simulink library "carnotUIBK_bus"  (R2023b)
settings: Solver=VariableStepAuto  StartTime=0.0  StopTime=10.0  RelTol=1e-3  EnableMultiTasking=on
values from neighbouring files (symbols this model uses):
  A = 7*10*2    (= 140)    [theta_ground_v1.m]    (also in xlswrite1.m = num2cell(data))
  amb_factor = 1    [DOOR.m]    (also in WALL.m; WINDOW.m = 0)
  area = obj.width * obj.height    [DOOR.m]    (also in RES.m = []; ROOM.m = 0; THERMALZONE.m = area + room(kk).area; WALL.m = area - obj.doors(jj).calc_area())
  B = A/(0.5 * P)    (= 8.23529411765)    [theta_ground_v1.m]
  boundary = BOUNDARY()    [BUILDING.m]    (also in WALL.m = '')
  building = obj    [BUILDING.m]    (also in create_building_automatic.m = building.save(); ini_building_automatic.m = building.add_variant_hvac(building.variant_hvac, hvac); load_building_automatic.m = building.save())
  C = zeros(1,length(d)+1)    [CONSTRUCTION.m]    (also in DOOR.m = [0 0 0]; WALL.m = [0 0 0]; WINDOW.m = [0 0 0])
  control = 2    [GAIN.m]    (also in GAINS.m)
  cp = str2num(value)    [CONSTRUCTION.m]
  height = 0    [DOOR.m]    (also in ROOM.m; THERMALZONE.m; WALL.m; WINDOW.m)
  p = [timevec_weather weather(:,12)]    [BOUNDARY.m]    (also in WEATHER.m = 0; init_carnotUIBK.m = cell2mat(carnotUIBKpaths(i,2)))
  rho = str2num(value)    [CONSTRUCTION.m]    (also in theta_ground_v1.m = 2000)
  type = 1    [CONSTRUCTION.m]    (also in GAINS.m = raw_moisture{ii,3}; STRUCTURE.m = 0)
  view_factor = 1    [DOOR.m]    (also in WINDOW.m = 0)
  wall = []    [ROOM.m]
  z = obj.Z    [WALL.m]    (also in theta_ground_v1.m = 0)
  zone = obj.zone(ind)    [THERMALZONE.m]
undefined symbols (not defined in the file or in its folder): const, Dd, get_building, mdot_air, mdot_CO2, mdot_H2O, mdot_VOC, pos, Qdot_C, Qdot_H, Qdot_I_electricity, Qdot_I_light, Qdot_I_person, Qdot_S, Qdot_T_ground, Qdot_T_internal, Qdot_T_neighbour, Qdot_T_opaque, Qdot_T_window, Qdot_V_infiltration, Qdot_V_mech, Qdot_V_window, Qdotc, Qdotr, r_frame, solar_ratio, solar_ratio1, solar_ratio2, Tc, Tr, Ts, Uvalue, wallsurface, window, window_height, window_heigth, window_width, windowsurface, x_CO2, x_H2O, x_VOC
libraries: $bdroot x134, carnot x87, simulink_extras x14, slpidlib x4, simulink x3
(part 5 of 12)

== system carnotUIBK_bus/HVAC/HVAC_9002_window opening/window opening 2 ==
  setpoint : Inport
  AIB : Inport  Port=2
  WDB : Inport  Port=3
  Enable : EnablePort
  Add : Sum
  Bus Selector1 : BusSelector  OutputSignals=Temperature_Ambient
  Bus Selector5 : BusSelector  OutputSignals=Ts,Tc,p,x_H2O
  Product : Product
  Saturation : Saturate  UpperLimit=1  LowerLimit=0
  Sum : Sum  Inputs=|-+
  Sum1 : Sum  Inputs=|+-
  Sum2 : Sum  Inputs=|-+
  Transfer Fcn (with initial states)1 : Subsystem  mask(Transfer Function with Initial States){N=[1], D=[600 1], X0=0}
      mask prompts: N "Numerator:"; D "Denominator:"; X0 "Initial conditions:"
      mask help: Vector expressions for numerator, and denominator. Coefficients are in descending powers of s.
      mask init:
      | [A,B,C,Dd]=tf2ss(N,D);if (isempty(X0));[m,n]=size(A);X0=zeros(1,m); end;
      mask Help: Specify the initial states for the transfer function.  The state ordering is determined by the m-file tf2ss.  There is no unique mapping of the states in a transfer function to states in a state-space representation.  However, tf2ss will consistently use the same mapping for a given transfer function.
      mask Display: dpoly(N,D,'s')
  Transfer Fcn (with initial states)2 : Subsystem  mask(Transfer Function with Initial States){N=[1], D=[600 1], X0=0}
      mask prompts: N "Numerator:"; D "Denominator:"; X0 "Initial conditions:"
      mask help: Vector expressions for numerator, and denominator. Coefficients are in descending powers of s.
      mask init:
      | [A,B,C,Dd]=tf2ss(N,D);if (isempty(X0));[m,n]=size(A);X0=zeros(1,m); end;
      mask Help: Specify the initial states for the transfer function.  The state ordering is determined by the m-file tf2ss.  There is no unique mapping of the states in a transfer function to states in a state-space representation.  However, tf2ss will consistently use the same mapping for a given transfer function.
      mask Display: dpoly(N,D,'s')
  Transfer Fcn (with initial states)3 : Subsystem  mask(Transfer Function with Initial States){N=[1], D=[600 1], X0=0}
      mask prompts: N "Numerator:"; D "Denominator:"; X0 "Initial conditions:"
      mask help: Vector expressions for numerator, and denominator. Coefficients are in descending powers of s.
      mask init:
      | [A,B,C,Dd]=tf2ss(N,D);if (isempty(X0));[m,n]=size(A);X0=zeros(1,m); end;
      mask Help: Specify the initial states for the transfer function.  The state ordering is determined by the m-file tf2ss.  There is no unique mapping of the states in a transfer function to states in a state-space representation.  However, tf2ss will consistently use the same mapping for a given transfer function.
      mask Display: dpoly(N,D,'s')
  on/off ambient : Relay  OnSwitchValue=0.5  OffSwitchValue=-0.5
  on/off hum : Relay  OnSwitchValue=0.5  OffSwitchValue=-0.5
  on/off roomtemp : Relay  OnSwitchValue=0.5  OffSwitchValue=-0.5
  setpoint humidity : Constant  Value=85
  x2RelHum_UIBK : carnot/Basic/Material_Properties/x2RelHum
      settings: SourceProductName=Carnot
  state : Outport  VectorParamsAs1DForOutWhenUnconnected=off
  wires:
  Transfer Fcn (with initial states)1/1(Out1) -> Sum2/2
  Transfer Fcn (with initial states)3/1(Out1) -> Sum1/2
  Transfer Fcn (with initial states)2/1(Out1) -> Sum/2, Sum1/1
  Saturation/1 -> state/1
  on/off hum/1 -> Add/1
  Product/1 -> Add/2
  Add/1 -> Saturation/1
  setpoint humidity/1 -> Sum2/1
  x2RelHum_UIBK/1 -> Transfer Fcn (with initial states)1/1(In1)
  Sum2/1 -> on/off hum/1
  Bus Selector5/4 -> x2RelHum_UIBK/3  "<x_H2O>"
  Bus Selector5/3 -> x2RelHum_UIBK/2  "<p>"
  Bus Selector5/2 -> x2RelHum_UIBK/1  "<Tc>"
  on/off ambient/1 -> Product/2
  Sum1/1 -> on/off ambient/1
  Bus Selector1/1 -> Transfer Fcn (with initial states)3/1(In1)  "<Temperature_Ambient>"
  WDB/1 -> Bus Selector1/1
  on/off roomtemp/1 -> Product/1
  Sum/1 -> on/off roomtemp/1
  Bus Selector5/1 -> Transfer Fcn (with initial states)2/1(In1)  "<Ts>"
  setpoint/1 -> Sum/1
  AIB/1 -> Bus Selector5/1

== system carnotUIBK_bus/HVAC/HVAC_9002_window opening/window opening 3 ==
  setpoint : Inport
  AIB : Inport  Port=2
  WDB : Inport  Port=3
  Enable : EnablePort
  Add : Sum
  Bus Selector1 : BusSelector  OutputSignals=Temperature_Ambient
  Bus Selector5 : BusSelector  OutputSignals=Ts,Tc,p,x_H2O
  Product : Product
  Saturation : Saturate  UpperLimit=1  LowerLimit=0
  Sum : Sum  Inputs=|-+
  Sum1 : Sum  Inputs=|+-
  Sum2 : Sum  Inputs=|-+
  Transfer Fcn (with initial states)1 : Subsystem  mask(Transfer Function with Initial States){N=[1], D=[600 1], X0=0}
      mask prompts: N "Numerator:"; D "Denominator:"; X0 "Initial conditions:"
      mask help: Vector expressions for numerator, and denominator. Coefficients are in descending powers of s.
      mask init:
      | [A,B,C,Dd]=tf2ss(N,D);if (isempty(X0));[m,n]=size(A);X0=zeros(1,m); end;
      mask Help: Specify the initial states for the transfer function.  The state ordering is determined by the m-file tf2ss.  There is no unique mapping of the states in a transfer function to states in a state-space representation.  However, tf2ss will consistently use the same mapping for a given transfer function.
      mask Display: dpoly(N,D,'s')
  Transfer Fcn (with initial states)2 : Subsystem  mask(Transfer Function with Initial States){N=[1], D=[600 1], X0=0}
      mask prompts: N "Numerator:"; D "Denominator:"; X0 "Initial conditions:"
      mask help: Vector expressions for numerator, and denominator. Coefficients are in descending powers of s.
      mask init:
      | [A,B,C,Dd]=tf2ss(N,D);if (isempty(X0));[m,n]=size(A);X0=zeros(1,m); end;
      mask Help: Specify the initial states for the transfer function.  The state ordering is determined by the m-file tf2ss.  There is no unique mapping of the states in a transfer function to states in a state-space representation.  However, tf2ss will consistently use the same mapping for a given transfer function.
      mask Display: dpoly(N,D,'s')
  Transfer Fcn (with initial states)3 : Subsystem  mask(Transfer Function with Initial States){N=[1], D=[600 1], X0=0}
      mask prompts: N "Numerator:"; D "Denominator:"; X0 "Initial conditions:"
      mask help: Vector expressions for numerator, and denominator. Coefficients are in descending powers of s.
      mask init:
      | [A,B,C,Dd]=tf2ss(N,D);if (isempty(X0));[m,n]=size(A);X0=zeros(1,m); end;
      mask Help: Specify the initial states for the transfer function.  The state ordering is determined by the m-file tf2ss.  There is no unique mapping of the states in a transfer function to states in a state-space representation.  However, tf2ss will consistently use the same mapping for a given transfer function.
      mask Display: dpoly(N,D,'s')
  on/off ambient : Relay  OnSwitchValue=0.5  OffSwitchValue=-0.5
  on/off hum : Relay  OnSwitchValue=0.5  OffSwitchValue=-0.5
  on/off roomtemp : Relay  OnSwitchValue=0.5  OffSwitchValue=-0.5
  setpoint humidity : Constant  Value=85
  x2RelHum_UIBK : carnot/Basic/Material_Properties/x2RelHum
      settings: SourceProductName=Carnot
  state : Outport  VectorParamsAs1DForOutWhenUnconnected=off
  wires:
  AIB/1 -> Bus Selector5/1
  setpoint/1 -> Sum/1
  Bus Selector5/1 -> Transfer Fcn (with initial states)3/1(In1)  "<Ts>"
  Sum/1 -> on/off roomtemp/1
  on/off roomtemp/1 -> Product/1
  WDB/1 -> Bus Selector1/1
  Bus Selector1/1 -> Transfer Fcn (with initial states)2/1(In1)  "<Temperature_Ambient>"
  Sum1/1 -> on/off ambient/1
  on/off ambient/1 -> Product/2
  Bus Selector5/2 -> x2RelHum_UIBK/1  "<Tc>"
  Bus Selector5/3 -> x2RelHum_UIBK/2  "<p>"
  Bus Selector5/4 -> x2RelHum_UIBK/3  "<x_H2O>"
  Sum2/1 -> on/off hum/1
  x2RelHum_UIBK/1 -> Transfer Fcn (with initial states)1/1(In1)
  setpoint humidity/1 -> Sum2/1
  Add/1 -> Saturation/1
  Product/1 -> Add/2
  on/off hum/1 -> Add/1
  Saturation/1 -> state/1
  Transfer Fcn (with initial states)3/1(Out1) -> Sum1/1, Sum/2
  Transfer Fcn (with initial states)2/1(Out1) -> Sum1/2
  Transfer Fcn (with initial states)1/1(Out1) -> Sum2/2

== system carnotUIBK_bus/HVAC/HVAC_9002_window opening/window opening 4 ==
  setpoint : Inport
  AIB : Inport  Port=2
  WDB : Inport  Port=3
  Enable : EnablePort
  Add : Sum
  Bus Selector1 : BusSelector  OutputSignals=Temperature_Ambient
  Bus Selector5 : BusSelector  OutputSignals=Ts,Tc,p,x_H2O
  Product : Product
  Saturation : Saturate  UpperLimit=1  LowerLimit=0
  Sum : Sum  Inputs=|-+
  Sum1 : Sum  Inputs=|+-
  Sum2 : Sum  Inputs=|-+
  Transfer Fcn (with initial states)1 : Subsystem  mask(Transfer Function with Initial States){N=[1], D=[600 1], X0=0}
      mask prompts: N "Numerator:"; D "Denominator:"; X0 "Initial conditions:"
      mask help: Vector expressions for numerator, and denominator. Coefficients are in descending powers of s.
      mask init:
      | [A,B,C,Dd]=tf2ss(N,D);if (isempty(X0));[m,n]=size(A);X0=zeros(1,m); end;
      mask Help: Specify the initial states for the transfer function.  The state ordering is determined by the m-file tf2ss.  There is no unique mapping of the states in a transfer function to states in a state-space representation.  However, tf2ss will consistently use the same mapping for a given transfer function.
      mask Display: dpoly(N,D,'s')
  Transfer Fcn (with initial states)2 : Subsystem  mask(Transfer Function with Initial States){N=[1], D=[600 1], X0=0}
      mask prompts: N "Numerator:"; D "Denominator:"; X0 "Initial conditions:"
      mask help: Vector expressions for numerator, and denominator. Coefficients are in descending powers of s.
      mask init:
      | [A,B,C,Dd]=tf2ss(N,D);if (isempty(X0));[m,n]=size(A);X0=zeros(1,m); end;
      mask Help: Specify the initial states for the transfer function.  The state ordering is determined by the m-file tf2ss.  There is no unique mapping of the states in a transfer function to states in a state-space representation.  However, tf2ss will consistently use the same mapping for a given transfer function.
      mask Display: dpoly(N,D,'s')
  Transfer Fcn (with initial states)3 : Subsystem  mask(Transfer Function with Initial States){N=[1], D=[600 1], X0=0}
      mask prompts: N "Numerator:"; D "Denominator:"; X0 "Initial conditions:"
      mask help: Vector expressions for numerator, and denominator. Coefficients are in descending powers of s.
      mask init:
      | [A,B,C,Dd]=tf2ss(N,D);if (isempty(X0));[m,n]=size(A);X0=zeros(1,m); end;
      mask Help: Specify the initial states for the transfer function.  The state ordering is determined by the m-file tf2ss.  There is no unique mapping of the states in a transfer function to states in a state-space representation.  However, tf2ss will consistently use the same mapping for a given transfer function.
      mask Display: dpoly(N,D,'s')
  on/off ambient : Relay  OnSwitchValue=0.5  OffSwitchValue=-0.5
  on/off hum : Relay  OnSwitchValue=0.5  OffSwitchValue=-0.5
  on/off roomtemp : Relay  OnSwitchValue=0.5  OffSwitchValue=-0.5
  setpoint humidity : Constant  Value=85
  x2RelHum_UIBK : carnot/Basic/Material_Properties/x2RelHum
      settings: SourceProductName=Carnot
  state : Outport  VectorParamsAs1DForOutWhenUnconnected=off
  wires:
  Transfer Fcn (with initial states)1/1(Out1) -> Sum2/2
  Transfer Fcn (with initial states)2/1(Out1) -> Sum1/2
  Transfer Fcn (with initial states)3/1(Out1) -> Sum/2, Sum1/1
  Saturation/1 -> state/1
  on/off hum/1 -> Add/1
  Product/1 -> Add/2
  Add/1 -> Saturation/1
  setpoint humidity/1 -> Sum2/1
  x2RelHum_UIBK/1 -> Transfer Fcn (with initial states)1/1(In1)
  Sum2/1 -> on/off hum/1
  Bus Selector5/4 -> x2RelHum_UIBK/3  "<x_H2O>"
  Bus Selector5/3 -> x2RelHum_UIBK/2  "<p>"
  Bus Selector5/2 -> x2RelHum_UIBK/1  "<Tc>"
  on/off ambient/1 -> Product/2
  Sum1/1 -> on/off ambient/1
  Bus Selector1/1 -> Transfer Fcn (with initial states)2/1(In1)  "<Temperature_Ambient>"
  WDB/1 -> Bus Selector1/1
  on/off roomtemp/1 -> Product/1
  Sum/1 -> on/off roomtemp/1
  Bus Selector5/1 -> Transfer Fcn (with initial states)3/1(In1)  "<Ts>"
  setpoint/1 -> Sum/1
  AIB/1 -> Bus Selector5/1

== system carnotUIBK_bus/HVAC/HVAC_9002_window opening/window opening 5 ==
  setpoint : Inport
  AIB : Inport  Port=2
  WDB : Inport  Port=3
  Enable : EnablePort
  Add : Sum
  Bus Selector1 : BusSelector  OutputSignals=Temperature_Ambient
  Bus Selector5 : BusSelector  OutputSignals=Ts,Tc,p,x_H2O
  Product : Product
  Saturation : Saturate  UpperLimit=1  LowerLimit=0
  Sum : Sum  Inputs=|-+
  Sum1 : Sum  Inputs=|+-
  Sum2 : Sum  Inputs=|-+
  Transfer Fcn (with initial states)1 : Subsystem  mask(Transfer Function with Initial States){N=[1], D=[600 1], X0=0}
      mask prompts: N "Numerator:"; D "Denominator:"; X0 "Initial conditions:"
      mask help: Vector expressions for numerator, and denominator. Coefficients are in descending powers of s.
      mask init:
      | [A,B,C,Dd]=tf2ss(N,D);if (isempty(X0));[m,n]=size(A);X0=zeros(1,m); end;
      mask Help: Specify the initial states for the transfer function.  The state ordering is determined by the m-file tf2ss.  There is no unique mapping of the states in a transfer function to states in a state-space representation.  However, tf2ss will consistently use the same mapping for a given transfer function.
      mask Display: dpoly(N,D,'s')
  Transfer Fcn (with initial states)2 : Subsystem  mask(Transfer Function with Initial States){N=[1], D=[600 1], X0=0}
      mask prompts: N "Numerator:"; D "Denominator:"; X0 "Initial conditions:"
      mask help: Vector expressions for numerator, and denominator. Coefficients are in descending powers of s.
      mask init:
      | [A,B,C,Dd]=tf2ss(N,D);if (isempty(X0));[m,n]=size(A);X0=zeros(1,m); end;
      mask Help: Specify the initial states for the transfer function.  The state ordering is determined by the m-file tf2ss.  There is no unique mapping of the states in a transfer function to states in a state-space representation.  However, tf2ss will consistently use the same mapping for a given transfer function.
      mask Display: dpoly(N,D,'s')
  Transfer Fcn (with initial states)3 : Subsystem  mask(Transfer Function with Initial States){N=[1], D=[600 1], X0=0}
      mask prompts: N "Numerator:"; D "Denominator:"; X0 "Initial conditions:"
      mask help: Vector expressions for numerator, and denominator. Coefficients are in descending powers of s.
      mask init:
      | [A,B,C,Dd]=tf2ss(N,D);if (isempty(X0));[m,n]=size(A);X0=zeros(1,m); end;
      mask Help: Specify the initial states for the transfer function.  The state ordering is determined by the m-file tf2ss.  There is no unique mapping of the states in a transfer function to states in a state-space representation.  However, tf2ss will consistently use the same mapping for a given transfer function.
      mask Display: dpoly(N,D,'s')
  on/off ambient : Relay  OnSwitchValue=0.5  OffSwitchValue=-0.5
  on/off hum : Relay  OnSwitchValue=0.5  OffSwitchValue=-0.5
  on/off roomtemp : Relay  OnSwitchValue=0.5  OffSwitchValue=-0.5
  setpoint humidity : Constant  Value=85
  x2RelHum_UIBK : carnot/Basic/Material_Properties/x2RelHum
      settings: SourceProductName=Carnot
  state : Outport  VectorParamsAs1DForOutWhenUnconnected=off
  wires:
  AIB/1 -> Bus Selector5/1
  setpoint/1 -> Sum/1
  Bus Selector5/1 -> Transfer Fcn (with initial states)2/1(In1)  "<Ts>"
  Sum/1 -> on/off roomtemp/1
  on/off roomtemp/1 -> Product/1
  WDB/1 -> Bus Selector1/1
  Bus Selector1/1 -> Transfer Fcn (with initial states)3/1(In1)  "<Temperature_Ambient>"
  Sum1/1 -> on/off ambient/1
  on/off ambient/1 -> Product/2
  Bus Selector5/2 -> x2RelHum_UIBK/1  "<Tc>"
  Bus Selector5/3 -> x2RelHum_UIBK/2  "<p>"
  Bus Selector5/4 -> x2RelHum_UIBK/3  "<x_H2O>"
  Sum2/1 -> on/off hum/1
  x2RelHum_UIBK/1 -> Transfer Fcn (with initial states)1/1(In1)
  setpoint humidity/1 -> Sum2/1
  Add/1 -> Saturation/1
  Product/1 -> Add/2
  on/off hum/1 -> Add/1
  Saturation/1 -> state/1
  Transfer Fcn (with initial states)2/1(Out1) -> Sum1/1, Sum/2
  Transfer Fcn (with initial states)3/1(Out1) -> Sum1/2
  Transfer Fcn (with initial states)1/1(Out1) -> Sum2/2

== system carnotUIBK_bus/HVAC/HVAC_9002_window opening/window opening 6 ==
  setpoint : Inport
  AIB : Inport  Port=2
  WDB : Inport  Port=3
  Enable : EnablePort
  Add : Sum
  Bus Selector1 : BusSelector  OutputSignals=Temperature_Ambient
  Bus Selector5 : BusSelector  OutputSignals=Ts,Tc,p,x_H2O
  Product : Product
  Saturation : Saturate  UpperLimit=1  LowerLimit=0
  Sum : Sum  Inputs=|-+
  Sum1 : Sum  Inputs=|+-
  Sum2 : Sum  Inputs=|-+
  Transfer Fcn (with initial states)1 : Subsystem  mask(Transfer Function with Initial States){N=[1], D=[600 1], X0=0}
      mask prompts: N "Numerator:"; D "Denominator:"; X0 "Initial conditions:"
      mask help: Vector expressions for numerator, and denominator. Coefficients are in descending powers of s.
      mask init:
      | [A,B,C,Dd]=tf2ss(N,D);if (isempty(X0));[m,n]=size(A);X0=zeros(1,m); end;
      mask Help: Specify the initial states for the transfer function.  The state ordering is determined by the m-file tf2ss.  There is no unique mapping of the states in a transfer function to states in a state-space representation.  However, tf2ss will consistently use the same mapping for a given transfer function.
      mask Display: dpoly(N,D,'s')
  Transfer Fcn (with initial states)2 : Subsystem  mask(Transfer Function with Initial States){N=[1], D=[600 1], X0=0}
      mask prompts: N "Numerator:"; D "Denominator:"; X0 "Initial conditions:"
      mask help: Vector expressions for numerator, and denominator. Coefficients are in descending powers of s.
      mask init:
      | [A,B,C,Dd]=tf2ss(N,D);if (isempty(X0));[m,n]=size(A);X0=zeros(1,m); end;
      mask Help: Specify the initial states for the transfer function.  The state ordering is determined by the m-file tf2ss.  There is no unique mapping of the states in a transfer function to states in a state-space representation.  However, tf2ss will consistently use the same mapping for a given transfer function.
      mask Display: dpoly(N,D,'s')
  Transfer Fcn (with initial states)3 : Subsystem  mask(Transfer Function with Initial States){N=[1], D=[600 1], X0=0}
      mask prompts: N "Numerator:"; D "Denominator:"; X0 "Initial conditions:"
      mask help: Vector expressions for numerator, and denominator. Coefficients are in descending powers of s.
      mask init:
      | [A,B,C,Dd]=tf2ss(N,D);if (isempty(X0));[m,n]=size(A);X0=zeros(1,m); end;
      mask Help: Specify the initial states for the transfer function.  The state ordering is determined by the m-file tf2ss.  There is no unique mapping of the states in a transfer function to states in a state-space representation.  However, tf2ss will consistently use the same mapping for a given transfer function.
      mask Display: dpoly(N,D,'s')
  on/off ambient : Relay  OnSwitchValue=0.5  OffSwitchValue=-0.5
  on/off hum : Relay  OnSwitchValue=0.5  OffSwitchValue=-0.5
  on/off roomtemp : Relay  OnSwitchValue=0.5  OffSwitchValue=-0.5
  setpoint humidity : Constant  Value=85
  x2RelHum_UIBK : carnot/Basic/Material_Properties/x2RelHum
      settings: SourceProductName=Carnot
  state : Outport  VectorParamsAs1DForOutWhenUnconnected=off
  wires:
  Transfer Fcn (with initial states)1/1(Out1) -> Sum2/2
  Transfer Fcn (with initial states)3/1(Out1) -> Sum1/2
  Transfer Fcn (with initial states)2/1(Out1) -> Sum/2, Sum1/1
  Saturation/1 -> state/1
  on/off hum/1 -> Add/1
  Product/1 -> Add/2
  Add/1 -> Saturation/1
  setpoint humidity/1 -> Sum2/1
  x2RelHum_UIBK/1 -> Transfer Fcn (with initial states)1/1(In1)
  Sum2/1 -> on/off hum/1
  Bus Selector5/4 -> x2RelHum_UIBK/3  "<x_H2O>"
  Bus Selector5/3 -> x2RelHum_UIBK/2  "<p>"
  Bus Selector5/2 -> x2RelHum_UIBK/1  "<Tc>"
  on/off ambient/1 -> Product/2
  Sum1/1 -> on/off ambient/1
  Bus Selector1/1 -> Transfer Fcn (with initial states)3/1(In1)  "<Temperature_Ambient>"
  WDB/1 -> Bus Selector1/1
  on/off roomtemp/1 -> Product/1
  Sum/1 -> on/off roomtemp/1
  Bus Selector5/1 -> Transfer Fcn (with initial states)2/1(In1)  "<Ts>"
  setpoint/1 -> Sum/1
  AIB/1 -> Bus Selector5/1

== system carnotUIBK_bus/HVAC/HVAC_999_TEMPLATE/Transfer Fcn (with initial states)1 ==
  In1 : Inport
  State Space : StateSpace  A=A  B=B  C=C  D=Dd  InitialCondition=X0
  Out1 : Outport  InitialOutput=0  VectorParamsAs1DForOutWhenUnconnected=off
  wires:
  In1/1 -> State Space/1
  State Space/1 -> Out1/1

== system carnotUIBK_bus/airexchange_intersection/airexchange_empiric/Subsystem ==
  note: (kg/s)
  note: (kg/s)
  note: (kg/s)
  note: (kg/kg)
  note: (kg/kg)
  note: ASSUMPTION: mdot_air_out2in = mdot_air_in2out !
  mdot_air : Inport
  x_in : Inport  Port=2
  x_out : Inport  Port=3
  Demux2 : Demux  Outputs=2
      settings: DisplayOption=none
  Demux3 : Demux  Outputs=2
      settings: DisplayOption=none
  Fcn{,1..3} (4 alike) : Fcn  Expr=u / (1+u)
  Product5 : Product  InputSameDT=on  SaturateOnIntegerOverflow=on  OutDataTypeStr=Inherit: Same as first input
  Product6 : Product  InputSameDT=on  SaturateOnIntegerOverflow=on  OutDataTypeStr=Inherit: Same as first input
  Sum1 : Sum  Inputs=+-  InputSameDT=on  SaturateOnIntegerOverflow=on  OutDataTypeStr=Inherit: Same as first input
  Sum2 : Sum  Inputs=+-  InputSameDT=on  SaturateOnIntegerOverflow=on  OutDataTypeStr=Inherit: Same as first input
  mdot_H2O : Outport  InitialOutput=0  VectorParamsAs1DForOutWhenUnconnected=off
  mdot_CO2 : Outport  Port=2  InitialOutput=0  VectorParamsAs1DForOutWhenUnconnected=off
  wires:
  x_out/1 -> Demux2/1
  Demux2/1 -> Fcn/1  "x_H2O_out"
  Demux2/2 -> Fcn1/1  "x_CO2_out"
  Demux3/2 -> Fcn3/1  "x_CO2_in"
  Demux3/1 -> Fcn2/1  "x_H2O_in"
  x_in/1 -> Demux3/1
  Fcn/1 -> Sum1/1
  Fcn2/1 -> Sum1/2
  Fcn1/1 -> Sum2/1
  Fcn3/1 -> Sum2/2
  Sum2/1 -> Product6/2
  Sum1/1 -> Product5/2
  mdot_air/1 -> Product6/1, Product5/1  "mdot_air >=0"
  Product6/1 -> mdot_CO2/1
  Product5/1 -> mdot_H2O/1

== system carnotUIBK_bus/airexchange_intersection/airexchange_empiric/V exchange ==
  Tc in : Inport
  x in : Inport  Port=2
  Tc out : Inport  Port=3
  x out : Inport  Port=4
  control : Inport  Port=5
  Abs : Abs  SaturateOnIntegerOverflow=off
  Gain1 : Gain  Gain=164.4
  Gain2 : Gain  Gain=32.6/164.4
  Gain4 : Gain  Gain=1000
  Gain5 : Gain  Gain=1000
  Product : Product
  Sum10 : Sum  InputSameDT=on  SaturateOnIntegerOverflow=on  OutDataTypeStr=Inherit: Same as first input
  Sum11 : Sum  Inputs=+-  InputSameDT=on  SaturateOnIntegerOverflow=on  OutDataTypeStr=Inherit: Same as first input
  Sum12 : Sum  Inputs=+-  InputSameDT=on  SaturateOnIntegerOverflow=on  OutDataTypeStr=Inherit: Same as first input
  Sum9 : Sum  InputSameDT=on  SaturateOnIntegerOverflow=on  OutDataTypeStr=Inherit: Same as first input
  "on/off " : Constant  Value=183
  V exchange : Outport  VectorParamsAs1DForOutWhenUnconnected=off
  wires:
  Sum12/1 -> Gain2/1
  Gain1/1 -> Sum10/2
  Abs/1 -> Gain1/1
  Sum9/1 -> Abs/1
  Gain2/1 -> Sum9/2
  "on/off "/1 -> Sum10/1
  Sum11/1 -> Sum9/1
  Tc out/1 -> Sum11/2
  x in/1 -> Gain4/1
  Tc in/1 -> Sum11/1
  x out/1 -> Gain5/1
  Sum10/1 -> Product/1
  Product/1 -> V exchange/1
  Gain4/1 -> Sum12/1
  Gain5/1 -> Sum12/2
  control/1 -> Product/2

== system carnotUIBK_bus/airexchange_intersection/airexchange_powerlaw/Subsystem ==
  note: (kg/s)
  note: (kg/s)
  note: (kg/s)
  note: (kg/kg)
  note: (kg/kg)
  note: ASSUMPTION: mdot_air_out2in = mdot_air_in2out !
  mdot_air : Inport
  x_in : Inport  Port=2
  x_out : Inport  Port=3
  Demux2 : Demux  Outputs=2
      settings: DisplayOption=none
  Demux3 : Demux  Outputs=2
      settings: DisplayOption=none
  Fcn{,1..3} (4 alike) : Fcn  Expr=u / (1+u)
  Product5 : Product  InputSameDT=on  SaturateOnIntegerOverflow=on  OutDataTypeStr=Inherit: Same as first input
  Product6 : Product  InputSameDT=on  SaturateOnIntegerOverflow=on  OutDataTypeStr=Inherit: Same as first input
  Sum1 : Sum  Inputs=+-  InputSameDT=on  SaturateOnIntegerOverflow=on  OutDataTypeStr=Inherit: Same as first input
  Sum2 : Sum  Inputs=+-  InputSameDT=on  SaturateOnIntegerOverflow=on  OutDataTypeStr=Inherit: Same as first input
  mdot_H2O : Outport  InitialOutput=0  VectorParamsAs1DForOutWhenUnconnected=off
  mdot_CO2 : Outport  Port=2  InitialOutput=0  VectorParamsAs1DForOutWhenUnconnected=off
  wires:
  x_out/1 -> Demux2/1
  Demux2/1 -> Fcn/1  "x_H2O_out"
  Demux2/2 -> Fcn1/1  "x_CO2_out"
  Demux3/2 -> Fcn3/1  "x_CO2_in"
  Demux3/1 -> Fcn2/1  "x_H2O_in"
  x_in/1 -> Demux3/1
  Fcn/1 -> Sum1/1
  Fcn2/1 -> Sum1/2
  Fcn1/1 -> Sum2/1
  Fcn3/1 -> Sum2/2
  Sum2/1 -> Product6/2
  Sum1/1 -> Product5/2
  mdot_air/1 -> Product6/1, Product5/1  "mdot_air >=0"
  Product6/1 -> mdot_CO2/1
  Product5/1 -> mdot_H2O/1

== system carnotUIBK_bus/airexchange_intersection/airexchange_powerlaw/door open ==
  H (height of the door [m]) : Inport
  rho_i : Inport  Port=2
  rho_j : Inport  Port=3
  L : Inport  Port=4
  control : Inport  Port=5
  Abs : Abs  SaturateOnIntegerOverflow=off
  Abs1 : Abs  SaturateOnIntegerOverflow=off
  Abs2 : Abs  SaturateOnIntegerOverflow=off
  Add : Sum
  Cd : Constant  Value=0.78
  Constant1 : Constant  Value=0.5
  Constant2 : Constant  Value=0.5
  Constant3 : Constant  Value=0.5
  Math Function : Math  Operator=pow  SignedPower=on
  Math Function1 : Math  Operator=pow  SignedPower=on
  Product : Product
  Product2 : Product  Inputs=3
  Product3 : Product
  Product6 : Product  Inputs=5
  d_rho : Sum  Inputs=+-
  g : Constant  Value=9.81
  mean : Gain  Gain=0.5
  sqrt(2)/2 : Gain  Gain=0.707106781
  m_dot_open_door : Outport  VectorParamsAs1DForOutWhenUnconnected=off
  wires:
  Product3/1 -> Product/2
  control/1 -> Product/1
  Product/1 -> m_dot_open_door/1
  d_rho/1 -> Product2/3
  Product2/1 -> Abs/1
  g/1 -> Product2/2
  Math Function/1 -> Product3/2
  Constant2/1 -> Math Function/2
  Abs/1 -> Math Function/1
  Product6/1 -> Abs2/1  "C_coeff"
  mean/1 -> Abs1/1
  sqrt(2)/2/1 -> Product6/1
  Add/1 -> mean/1
  H (height of the door [m])/1 -> Product2/1, Product6/3
  rho_j/1 -> Add/2, d_rho/2
  rho_i/1 -> d_rho/1, Add/1
  L/1 -> Product6/2
  Cd/1 -> sqrt(2)/2/1
  Constant1/1 -> Product6/5
  Constant3/1 -> Math Function1/2
  Abs1/1 -> Math Function1/1
  Math Function1/1 -> Product6/4
  Abs2/1 -> Product3/1

== system carnotUIBK_bus/gain/Equipment/W//device ==
  Switch : Inport
  Bus Assignment2 : BusAssignment  AssignedSignals=Qdotc,Qdotr,Qdot_I_electricity
  Gain1 : Gain  Gain=0.6  SaturateOnIntegerOverflow=on  OutDataTypeStr=Inherit: Same as input  ParamDataTypeStr=Inherit: Same as input
  Gain4 : Gain  Gain=0.4  SaturateOnIntegerOverflow=on  OutDataTypeStr=Inherit: Same as input  ParamDataTypeStr=Inherit: Same as input
  Profile W/device : carnot/Load/General/Repeating_Profile  period=timevalues(end)  rep_seq_t=timevalues(1:end-1)  rep_seq_d=timeduration  rep_seq_y=values1
      settings: SourceProductName=Carnot
  S_initialize : $bdroot/general/S_initialize  SystemSampleTime=-1  VariantActivationTime=update diagram  AllowFlexibleInterface=on  Latency=0  AutoFrameSizeCalculation=off
  Switch3 : Switch  Criteria=u2 > Threshold  SaturateOnIntegerOverflow=off  InputSameDT=off
  timeconstant : simulink_extras/Additional Linear/Transfer Fcn (with initial outputs)  N=[1]  D=[60 1]  Y0=0  U0=0
  "[S]" : Outport  VectorParamsAs1DForOutWhenUnconnected=off
  wires:
  Gain4/1 -> Bus Assignment2/3
  Gain1/1 -> Bus Assignment2/2
  Profile W/device/1 -> timeconstant/1
  timeconstant/1 -> Gain4/1, Bus Assignment2/4, Gain1/1
  Switch/1 -> Switch3/2
  S_initialize/1 -> Switch3/3, Bus Assignment2/1
  Bus Assignment2/1 -> Switch3/1
  Switch3/1 -> "[S]"/1

== system carnotUIBK_bus/gain/Equipment/W//m² ==
  Switch : Inport
  Bus Assignment2 : BusAssignment  AssignedSignals=Qdotc,Qdotr,Qdot_I_electricity
  Gain1 : Gain  Gain=z.heated_area  SaturateOnIntegerOverflow=on  OutDataTypeStr=Inherit: Same as input  ParamDataTypeStr=Inherit: Same as input
  Gain3 : Gain  Gain=0.6  SaturateOnIntegerOverflow=on  OutDataTypeStr=Inherit: Same as input  ParamDataTypeStr=Inherit: Same as input
  Gain5 : Gain  Gain=0.4  SaturateOnIntegerOverflow=on  OutDataTypeStr=Inherit: Same as input  ParamDataTypeStr=Inherit: Same as input
  Profile W/m² : carnot/Load/General/Repeating_Profile  period=timevalues(end)  rep_seq_t=timevalues(1:end-1)  rep_seq_d=timeduration  rep_seq_y=values1
      settings: SourceProductName=Carnot
  S_initialize : $bdroot/general/S_initialize  SystemSampleTime=-1  VariantActivationTime=update diagram  AllowFlexibleInterface=on  Latency=0  AutoFrameSizeCalculation=off
  Switch3 : Switch  Criteria=u2 > Threshold  SaturateOnIntegerOverflow=off  InputSameDT=off
  timeconstant : simulink_extras/Additional Linear/Transfer Fcn (with initial outputs)  N=[1]  D=[60 1]  Y0=0  U0=0
  "[S]" : Outport  VectorParamsAs1DForOutWhenUnconnected=off
  wires:
  Gain5/1 -> Bus Assignment2/3
  Gain3/1 -> Bus Assignment2/2
  Profile W/m²/1 -> Gain1/1
  Gain1/1 -> timeconstant/1
  timeconstant/1 -> Bus Assignment2/4, Gain5/1, Gain3/1
  Switch/1 -> Switch3/2
  S_initialize/1 -> Switch3/3, Bus Assignment2/1
  Bus Assignment2/1 -> Switch3/1
  Switch3/1 -> "[S]"/1

== system carnotUIBK_bus/gain/Light/W//light ==
  Switch : Inport
  Bus Assignment2 : BusAssignment  AssignedSignals=Qdotc,Qdotr,Qdot_I_light
  Gain1 : Gain  Gain=0.6  SaturateOnIntegerOverflow=on  OutDataTypeStr=Inherit: Same as input  ParamDataTypeStr=Inherit: Same as input
  Gain4 : Gain  Gain=0.4  SaturateOnIntegerOverflow=on  OutDataTypeStr=Inherit: Same as input  ParamDataTypeStr=Inherit: Same as input
  Profile W/light : carnot/Load/General/Repeating_Profile  period=timevalues(end)  rep_seq_t=timevalues(1:end-1)  rep_seq_d=timeduration  rep_seq_y=values1
      settings: SourceProductName=Carnot
  S_initialize : $bdroot/general/S_initialize  SystemSampleTime=-1  VariantActivationTime=update diagram  AllowFlexibleInterface=on  Latency=0  AutoFrameSizeCalculation=off
  Switch3 : Switch  Criteria=u2 > Threshold  SaturateOnIntegerOverflow=off  InputSameDT=off
  timeconstant : simulink_extras/Additional Linear/Transfer Fcn (with initial outputs)  N=[1]  D=[60 1]  Y0=0  U0=0
  "[S]" : Outport  VectorParamsAs1DForOutWhenUnconnected=off
  wires:
  Gain4/1 -> Bus Assignment2/3
  Gain1/1 -> Bus Assignment2/2
  Profile W/light/1 -> timeconstant/1
  timeconstant/1 -> Bus Assignment2/4, Gain4/1, Gain1/1
  Switch/1 -> Switch3/2
  S_initialize/1 -> Switch3/3, Bus Assignment2/1
  Bus Assignment2/1 -> Switch3/1
  Switch3/1 -> "[S]"/1

== system carnotUIBK_bus/gain/Light/W//m² ==
  Switch : Inport
  Bus Assignment2 : BusAssignment  AssignedSignals=Qdotc,Qdotr,Qdot_I_light
  Gain1 : Gain  Gain=z.heated_area  SaturateOnIntegerOverflow=on  OutDataTypeStr=Inherit: Same as input  ParamDataTypeStr=Inherit: Same as input
  Gain3 : Gain  Gain=0.6  SaturateOnIntegerOverflow=on  OutDataTypeStr=Inherit: Same as input  ParamDataTypeStr=Inherit: Same as input
  Gain5 : Gain  Gain=0.4  SaturateOnIntegerOverflow=on  OutDataTypeStr=Inherit: Same as input  ParamDataTypeStr=Inherit: Same as input
  Profile W/m² : carnot/Load/General/Repeating_Profile  period=timevalues(end)  rep_seq_t=timevalues(1:end-1)  rep_seq_d=timeduration  rep_seq_y=values1
      settings: SourceProductName=Carnot
  S_initialize : $bdroot/general/S_initialize  SystemSampleTime=-1  VariantActivationTime=update diagram  AllowFlexibleInterface=on  Latency=0  AutoFrameSizeCalculation=off
  Switch3 : Switch  Criteria=u2 > Threshold  SaturateOnIntegerOverflow=off  InputSameDT=off
  timeconstant : simulink_extras/Additional Linear/Transfer Fcn (with initial outputs)  N=[1]  D=[60 1]  Y0=0  U0=0
  "[S]" : Outport  VectorParamsAs1DForOutWhenUnconnected=off
  wires:
  Gain5/1 -> Bus Assignment2/3
  Gain3/1 -> Bus Assignment2/2
  Profile W/m²/1 -> Gain1/1
  Gain1/1 -> timeconstant/1
  timeconstant/1 -> Gain5/1, Bus Assignment2/4, Gain3/1
  Switch/1 -> Switch3/2
  S_initialize/1 -> Switch3/3, Bus Assignment2/1
  Bus Assignment2/1 -> Switch3/1
  Switch3/1 -> "[S]"/1

== system carnotUIBK_bus/gain/Moisture/kg//s ==
  note: 2500 kJ/kg
  Bus Assignment2 : BusAssignment  AssignedSignals=Qdotc,Qdotr,mdot_H2O,Qdot_I_electricity
  Gain1 : Gain  Gain=1.0  SaturateOnIntegerOverflow=on  OutDataTypeStr=Inherit: Same as input  ParamDataTypeStr=Inherit: Same as input
  Gain2 : Gain  Gain=-2500000  SaturateOnIntegerOverflow=on  OutDataTypeStr=Inherit: Same as input  ParamDataTypeStr=Inherit: Same as input
  Gain4 : Gain  Gain=0.0  SaturateOnIntegerOverflow=on  OutDataTypeStr=Inherit: Same as input  ParamDataTypeStr=Inherit: Same as input
  Profile kg/s : carnot/Load/General/Repeating_Profile  period=timevalues(end)  rep_seq_t=timevalues(1:end-1)  rep_seq_d=timeduration  rep_seq_y=values1
      settings: SourceProductName=Carnot
  S_initialize : $bdroot/general/S_initialize  SystemSampleTime=-1  VariantActivationTime=update diagram  AllowFlexibleInterface=on  Latency=0  AutoFrameSizeCalculation=off
  timeconstant : simulink_extras/Additional Linear/Transfer Fcn (with initial outputs)  N=[1]  D=[60 1]  Y0=0  U0=0
  "[S]" : Outport  VectorParamsAs1DForOutWhenUnconnected=off
  wires:
  Gain4/1 -> Bus Assignment2/3
  Bus Assignment2/1 -> "[S]"/1
  Gain1/1 -> Bus Assignment2/2
  Profile kg/s/1 -> timeconstant/1
  Gain2/1 -> Gain4/1, Bus Assignment2/5, Gain1/1
  timeconstant/1 -> Bus Assignment2/4, Gain2/1
  S_initialize/1 -> Bus Assignment2/1

== system carnotUIBK_bus/gain/People/W//m² ==
  Switch : Inport
  Bus Assignment2 : BusAssignment  AssignedSignals=Qdotc,Qdotr,Qdot_I_person
  Gain1 : Gain  Gain=z.heated_area  SaturateOnIntegerOverflow=on  OutDataTypeStr=Inherit: Same as input  ParamDataTypeStr=Inherit: Same as input
  Gain2 : Gain  Gain=0.5  SaturateOnIntegerOverflow=on  OutDataTypeStr=Inherit: Same as input  ParamDataTypeStr=Inherit: Same as input
  Gain4 : Gain  Gain=0.5  SaturateOnIntegerOverflow=on  OutDataTypeStr=Inherit: Same as input  ParamDataTypeStr=Inherit: Same as input
  S_initialize : $bdroot/general/S_initialize  SystemSampleTime=-1  VariantActivationTime=update diagram  AllowFlexibleInterface=on  Latency=0  AutoFrameSizeCalculation=off
  Switch3 : Switch  Criteria=u2 > Threshold  SaturateOnIntegerOverflow=off  InputSameDT=off
  profile_1 : carnot/Load/General/Repeating_Profile  period=timevalues(end)  rep_seq_t=timevalues(1:end-1)  rep_seq_d=timeduration  rep_seq_y=values1
      settings: SourceProductName=Carnot
  timeconstant : simulink_extras/Additional Linear/Transfer Fcn (with initial outputs)  N=[1]  D=[60 1]  Y0=0  U0=0
  "[S]" : Outport  VectorParamsAs1DForOutWhenUnconnected=off
  wires:
  Gain1/1 -> timeconstant/1
  Gain4/1 -> Bus Assignment2/3
  Gain2/1 -> Bus Assignment2/2
  profile_1/1 -> Gain1/1
  timeconstant/1 -> Bus Assignment2/4, Gain4/1, Gain2/1
  Switch/1 -> Switch3/2
  S_initialize/1 -> Switch3/3, Bus Assignment2/1
  Bus Assignment2/1 -> Switch3/1
  Switch3/1 -> "[S]"/1

== system carnotUIBK_bus/gain/People/W//ppl (activity) ==
  Top : Inport
  Switch : Inport  Port=2
  Bus Assignment2 : BusAssignment  AssignedSignals=Qdotc,Qdotr,mdot_H2O,mdot_CO2,Qdot_I_person
  Gain1 : Gain  Gain=0.5  SaturateOnIntegerOverflow=on  OutDataTypeStr=Inherit: Same as input  ParamDataTypeStr=Inherit: Same as input
  Gain2 : Gain  Gain=0.5  SaturateOnIntegerOverflow=on  OutDataTypeStr=Inherit: Same as input  ParamDataTypeStr=Inherit: Same as input
  Gain4 : Gain  Gain=0.5  SaturateOnIntegerOverflow=on  OutDataTypeStr=Inherit: Same as input  ParamDataTypeStr=Inherit: Same as input
  LUT_Qdot_dry : Subsystem
      mask help:
      | This block delivers the SENSITIVE/DRY HEAT POWER one person emitts in a room depending on his activity and the actual sensitive temperature in the middle of a room.
      |
      | Qdot_dry	: sensitive/dry heat power emitted from 1 person, W
      | activity		: number of class of person activity (DIN 1946, VDI 2078):
      | 		   0 - no physical work (sleeping)
      | 		   1 - relaxed work (home, office, school)
      | 		   2 - light physical work, standing (shopping, laboratory)
      | 		   3 - moderately heavy physical activity (home work)
      | 		   4 - heavy physical activity (sports, heavy maschinery)
      | Top		: sensitive/operational temperature in the middle of a
      | 	  	  room/zone,°C
  LUT_Qdot_hum1 : Subsystem  mask(LOOK UP TABLE){}
      mask help:
      | This block delivers the LATENT/HUMID HEAT POWER one person emitts in a room depending on his activity and the actual sensitive temperature in the middle of a room.
      |
      | Qdot_hum	: latent/humid heat power emitted from 1 person, W
      | activity		: number of class of person activity (DIN 1946, VDI 2078):
      | 		   0 - no physical work (sleeping)
      | 		   1 - relaxed work (home, office, school)
      | 		   2 - light physical work standing (shopping, laboratory)
      | 		   3 - moderately heavy physical activity (home work)
      | 		   4 - heavy physical activity (sports, heavy maschinery)
      | Top		: sensitive/operational temperature in the middle of a
      | 		  room/zone,°C
  LUT_mdot_CO2 : Subsystem  mask(LOOK UP TABLE){}
      mask help:
      | This block delivers the CO2 MASS FLOW one person emitts in a room depending on his activity and the actual sensitive temperature in the middle of a room.
      |
      | mdot_CO2	: CO2 mass flow emitted from 1 person, kg/s
      | activity		: number of class of person activity (DIN 1946, VDI 2078):
      | 		   0 - no physical work (sleeping)
      | 		   1 - relaxed work (home, office, school)
      | 		   2 - light physical work standing (shopping, laboratory)
      | 		   3 - moderately heavy physical activity (home work)
      | 		   4 - heavy physical activity (sports, heavy maschinery)
  LUT_mdot_H2O : Subsystem  mask(LOOK UP TABLE){}
      mask help:
      | This block delivers the WATER MASS FLOW one person emitts in a room depending on his activity and the actual sensitive temperature in the middle of a room.
      |
      | mdot_H2O	: water mass flow emitted from 1 person, kg/s
      | activity		: number of class of person activity (DIN 1946, VDI 2078):
      | 		   0 - no physical work (sleeping)
      | 		   1 - relaxed work (home, office, school)
      | 		   2 - light physical work standing (shopping, laboratory)
      | 		   3 - moderately heavy physical activity (home work)
      | 		   4 - heavy physical activity (sports, heavy maschinery)
      | Top		: sensitive/operational temperature in the middle of a
      | 		  room/zone,°C
  Product{,2..4} (4 alike) : Product
  S_initialize : $bdroot/general/S_initialize  SystemSampleTime=-1  VariantActivationTime=update diagram  AllowFlexibleInterface=on  Latency=0  AutoFrameSizeCalculation=off
  Sum : Sum  InputSameDT=on  SaturateOnIntegerOverflow=on  OutDataTypeStr=Inherit: Same as first input
  Sum1 : Sum  InputSameDT=on  SaturateOnIntegerOverflow=on  OutDataTypeStr=Inherit: Same as first input
  Switch3 : Switch  Criteria=u2 > Threshold  SaturateOnIntegerOverflow=off  InputSameDT=off
  profile people : carnot/Load/General/Repeating_Profile  period=timevalues(end)  rep_seq_t=timevalues(1:end-1)  rep_seq_d=timeduration  rep_seq_y=values1
      settings: SourceProductName=Carnot
  profile people activity : carnot/Load/General/Repeating_Profile  period=timevalues(end)  rep_seq_t=timevalues(1:end-1)  rep_seq_d=timeduration  rep_seq_y=values2
      settings: SourceProductName=Carnot
  timeconstant{,1..3} (4 alike) : simulink_extras/Additional Linear/Transfer Fcn (with initial outputs)  N=[1]  D=[60 1]  Y0=0  U0=0
  "[S]" : Outport  VectorParamsAs1DForOutWhenUnconnected=off
  wires:
  Top/1 -> LUT_mdot_H2O/2(Top), LUT_Qdot_hum1/2(Top), LUT_Qdot_dry/2(Top)
  Switch3/1 -> "[S]"/1
  LUT_Qdot_dry/1(Qdot_dry) -> Product2/2
  Product3/1 -> timeconstant1/1  "mdot_H2O"
  Gain4/1 -> Bus Assignment2/3, Sum/2  "Qdot_r"
  Product4/1 -> timeconstant/1
  Sum/1 -> Bus Assignment2/2  "Qdot_c"
  LUT_Qdot_hum1/1(Qdot_hum) -> Product/2
  profile people activity/1 -> LUT_mdot_CO2/1(activity), LUT_mdot_H2O/1(activity), LUT_Qdot_dry/1(activity), LUT_Qdot_hum1/1(activity)
  Gain1/1 -> Sum1/1, Sum/1
  Gain2/1 -> Sum1/2, Gain4/1
  profile people/1 -> Product4/1, Product3/1, Product2/1, Product/1
  Product/1 -> timeconstant3/1
  Product2/1 -> timeconstant2/1
  LUT_mdot_CO2/1(mdot_CO2) -> Product4/2
  LUT_mdot_H2O/1(mdot_H2O) -> Product3/2
  timeconstant/1 -> Bus Assignment2/5
  timeconstant1/1 -> Bus Assignment2/4
  timeconstant2/1 -> Gain2/1
  timeconstant3/1 -> Gain1/1
  S_initialize/1 -> Switch3/3, Bus Assignment2/1
  Sum1/1 -> Bus Assignment2/6
  Switch/1 -> Switch3/2
  Bus Assignment2/1 -> Switch3/1

== system carnotUIBK_bus/gain/People/W//ppl (constant) ==
  Top : Inport
  Switch : Inport  Port=2
  Bus Assignment2 : BusAssignment  AssignedSignals=Qdotc,Qdotr,mdot_H2O,mdot_CO2,Qdot_I_person
  Gain1 : Gain  Gain=10  SaturateOnIntegerOverflow=on  OutDataTypeStr=Inherit: Same as input  ParamDataTypeStr=Inherit: Same as input
  Gain2 : Gain  Gain=50  SaturateOnIntegerOverflow=on  OutDataTypeStr=Inherit: Same as input  ParamDataTypeStr=Inherit: Same as input
  Gain4 : Gain  Gain=0.5  SaturateOnIntegerOverflow=on  OutDataTypeStr=Inherit: Same as input  ParamDataTypeStr=Inherit: Same as input
  LUT_mdot_CO2 : Subsystem  mask(LOOK UP TABLE){}
      mask help:
      | This block delivers the CO2 MASS FLOW one person emitts in a room depending on his activity and the actual sensitive temperature in the middle of a room.
      |
      | mdot_CO2	: CO2 mass flow emitted from 1 person, kg/s
      | activity		: number of class of person activity (DIN 1946, VDI 2078):
      | 		   0 - no physical work (sleeping)
      | 		   1 - relaxed work (home, office, school)
      | 		   2 - light physical work standing (shopping, laboratory)
      | 		   3 - moderately heavy physical activity (home work)
      | 		   4 - heavy physical activity (sports, heavy maschinery)
  LUT_mdot_H2O : Subsystem  mask(LOOK UP TABLE){}
      mask help:
      | This block delivers the WATER MASS FLOW one person emitts in a room depending on his activity and the actual sensitive temperature in the middle of a room.
      |
      | mdot_H2O	: water mass flow emitted from 1 person, kg/s
      | activity		: number of class of person activity (DIN 1946, VDI 2078):
      | 		   0 - no physical work (sleeping)
      | 		   1 - relaxed work (home, office, school)
      | 		   2 - light physical work standing (shopping, laboratory)
      | 		   3 - moderately heavy physical activity (home work)
      | 		   4 - heavy physical activity (sports, heavy maschinery)
      | Top		: sensitive/operational temperature in the middle of a
      | 		  room/zone,°C
  Product3 : Product
  Product4 : Product
  S_initialize : $bdroot/general/S_initialize  SystemSampleTime=-1  VariantActivationTime=update diagram  AllowFlexibleInterface=on  Latency=0  AutoFrameSizeCalculation=off
  Sum : Sum  InputSameDT=on  SaturateOnIntegerOverflow=on  OutDataTypeStr=Inherit: Same as first input
  Sum1 : Sum  InputSameDT=on  SaturateOnIntegerOverflow=on  OutDataTypeStr=Inherit: Same as first input
  Switch3 : Switch  Criteria=u2 > Threshold  SaturateOnIntegerOverflow=off  InputSameDT=off
  profile people : carnot/Load/General/Repeating_Profile  period=timevalues(end)  rep_seq_t=timevalues(1:end-1)  rep_seq_d=timeduration  rep_seq_y=values1
      settings: SourceProductName=Carnot
  profile people activity : carnot/Load/General/Repeating_Profile  period=timevalues(end)  rep_seq_t=timevalues(1:end-1)  rep_seq_d=timeduration  rep_seq_y=values2
      settings: SourceProductName=Carnot
  timeconstant{,1..3} (4 alike) : simulink_extras/Additional Linear/Transfer Fcn (with initial outputs)  N=[1]  D=[60 1]  Y0=0  U0=0
  "[S]" : Outport  VectorParamsAs1DForOutWhenUnconnected=off
  wires:
  Switch3/1 -> "[S]"/1
  Switch/1 -> Switch3/2
  Top/1 -> LUT_mdot_H2O/2(Top)
  Sum1/1 -> Bus Assignment2/6
  profile people/1 -> Product4/1, Product3/1, Gain2/1, Gain1/1
  Product3/1 -> timeconstant/1  "mdot_H2O"
  Gain4/1 -> Sum/2, Bus Assignment2/3  "Qdot_r"
  Product4/1 -> timeconstant1/1
  Sum/1 -> Bus Assignment2/2  "Qdot_c"
  Bus Assignment2/1 -> Switch3/1
  Gain1/1 -> timeconstant3/1
  Gain2/1 -> timeconstant2/1
  profile people activity/1 -> LUT_mdot_CO2/1(activity), LUT_mdot_H2O/1(activity)
  LUT_mdot_H2O/1(mdot_H2O) -> Product3/2  "mdot_H2O"
  LUT_mdot_CO2/1(mdot_CO2) -> Product4/2
  timeconstant/1 -> Bus Assignment2/4
  timeconstant1/1 -> Bus Assignment2/5
  timeconstant2/1 -> Gain4/1, Sum1/2
  timeconstant3/1 -> Sum/1, Sum1/1
  S_initialize/1 -> Switch3/3, Bus Assignment2/1

== system carnotUIBK_bus/infiltration/infiltration_constant/Subsystem ==
  note: ASSUMPTION: mdot_air_out2in = mdot_air_in2out !
  note: (kg/kg)
  note: (kg/kg)
  note: (kg/s)
  note: (kg/s)
  note: (kg/s)
  mdot_air : Inport
  x_in : Inport  Port=2
  x_out : Inport  Port=3
  Demux2 : Demux  Outputs=2
      settings: DisplayOption=none
  Demux3 : Demux  Outputs=2
      settings: DisplayOption=none
  Fcn{,1..3} (4 alike) : Fcn  Expr=u / (1+u)
  Product5 : Product  InputSameDT=on  SaturateOnIntegerOverflow=on  OutDataTypeStr=Inherit: Same as first input
  Product6 : Product  InputSameDT=on  SaturateOnIntegerOverflow=on  OutDataTypeStr=Inherit: Same as first input
  Sum1 : Sum  Inputs=+-  InputSameDT=on  SaturateOnIntegerOverflow=on  OutDataTypeStr=Inherit: Same as first input
  Sum2 : Sum  Inputs=+-  InputSameDT=on  SaturateOnIntegerOverflow=on  OutDataTypeStr=Inherit: Same as first input
  mdot_H2O : Outport  InitialOutput=0  VectorParamsAs1DForOutWhenUnconnected=off
  mdot_CO2 : Outport  Port=2  InitialOutput=0  VectorParamsAs1DForOutWhenUnconnected=off
  wires:
  Product5/1 -> mdot_H2O/1
  Product6/1 -> mdot_CO2/1
  mdot_air/1 -> Product5/1, Product6/1  "mdot_air >=0"
  Sum1/1 -> Product5/2
  Sum2/1 -> Product6/2
  Fcn3/1 -> Sum2/2
  Fcn1/1 -> Sum2/1
  Fcn2/1 -> Sum1/2
  Fcn/1 -> Sum1/1
  x_in/1 -> Demux3/1
  Demux3/1 -> Fcn2/1  "x_H2O_in"
  Demux3/2 -> Fcn3/1  "x_CO2_in"
  Demux2/2 -> Fcn1/1  "x_CO2_out"
  Demux2/1 -> Fcn/1  "x_H2O_out"
  x_out/1 -> Demux2/1

== system carnotUIBK_bus/infiltration/infiltration_constant/Window_Ventilation ==
  Troom : Inport
  Tamb : Inport  Port=2
  control : Inport  Port=3
  Mux : Mux  Inputs=3
  S-Function : S-Function  FunctionName=tiltvent  Parameters=alpha, H, W  SFunctionDeploymentMode=off  EnableBusSupport=off
  V_rate [m^3/s] : Outport  VectorParamsAs1DForOutWhenUnconnected=off
  wires:
  Troom/1 -> Mux/1
  Mux/1 -> S-Function/1
  S-Function/1 -> V_rate [m^3/s]/1
  control/1 -> Mux/3
  Tamb/1 -> Mux/2

== system carnotUIBK_bus/infiltration/infiltration_pressure/infiltration_pressure ==
  T_room : Inport
  WDB : Inport  Port=2
  H_window : Inport  Port=3
  facade_angle : Inport  Port=4
  add_coeff_wind : Inport  Port=5
  Add : Sum
  Bus Selector : BusSelector  OutputSignals=Temperature_Ambient,Station_Pressure,Wind_Speed,Wind_Direction
  Divide : Product  Inputs=*//
  Divide1 : Product  Inputs=**/
  K : Constant  Value=273.15
  Ra : Constant  Value=287.058
  dP_infiltration : Subsystem
  delta_p : Constant  Value=50
  n : Constant  Value=0.66
  n50 : Constant  Value=n50
  pow_law : Math  Operator=pow  SignedPower=on
  power_law_infiltration : Subsystem
  volume : Constant  Value=volume
  m_dot : Outport  VectorParamsAs1DForOutWhenUnconnected=off
  wires:
  power_law_infiltration/1(m_dot) -> m_dot/1
  dP_infiltration/1(dP_total) -> power_law_infiltration/1(dP)
  T_room/1 -> dP_infiltration/1(T_int)
  WDB/1 -> Bus Selector/1
  Bus Selector/1 -> Add/1, dP_infiltration/2(T_ext)  "<Temperature_Ambient>"
  Bus Selector/3 -> dP_infiltration/3(windspeed)  "<Wind_Speed>"
  Bus Selector/4 -> dP_infiltration/4(wind_angle)  "<Wind_Direction>"
  Bus Selector/2 -> Divide/1  "<Station_Pressure>"
  H_window/1 -> dP_infiltration/6(H_window)
  Ra/1 -> Divide/2
  K/1 -> Add/2
  Add/1 -> Divide/3
  n/1 -> power_law_infiltration/3(n), pow_law/2
  Divide/1 -> power_law_infiltration/4(density), dP_infiltration/5(air_density_ext)
  facade_angle/1 -> dP_infiltration/8(facade_angle)
  add_coeff_wind/1 -> dP_infiltration/7(add_coeff_wind)
  Divide1/1 -> power_law_infiltration/2(C)
  n50/1 -> Divide1/1
  pow_law/1 -> Divide1/3
  delta_p/1 -> pow_law/1
  volume/1 -> Divide1/2
